simulink library "tangentialToGroundPosition"  (R2020a)
settings: Solver=VariableStepAuto  StartTime=0.0  StopTime=10.0  RelTol=1e-3
libraries: rotationFromGroundToTangent x1
settings Model: Creator=Ayaz  LastModifiedBy=Ayaz

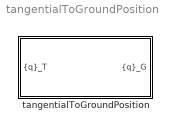
== system tangentialToGroundPosition ==
  tangentialToGroundPosition : Subsystem

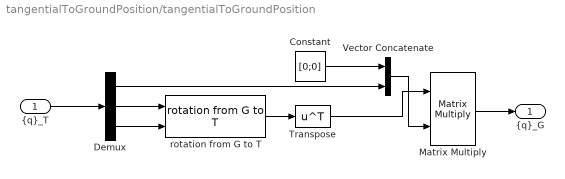
== system tangentialToGroundPosition/tangentialToGroundPosition ==
  "{q}_T" : Inport  PortDimensions=[3,1]
  Constant : Constant  Value=[0;0]  VectorParams1D=off
  Demux : Demux  Outputs=3
  Matrix Multiply : Product  Multiplication=Matrix(*)
  Transpose : Math  Operator=transpose  SaturateOnIntegerOverflow=on
  Vector Concatenate : Concatenate
  rotation from G to T : rotationFromGroundToTangent/rotation from G to T  SystemSampleTime=-1  Latency=0  AutoFrameSizeCalculation=off
  "{q}_G" : Outport
  wires:
  "{q}_T"/1 -> Demux/1
  Demux/2 -> rotation from G to T/1
  Demux/3 -> rotation from G to T/2
  rotation from G to T/1 -> Transpose/1
  Demux/1 -> Vector Concatenate/2
  Constant/1 -> Vector Concatenate/1
  Transpose/1 -> Matrix Multiply/1
  Vector Concatenate/1 -> Matrix Multiply/2
  Matrix Multiply/1 -> "{q}_G"/1
